simulink model "model1_visualize_video"  (R2025a)
settings: Solver=VariableStepAuto  StartTime=0.0  StopTime=10.0  RelTol=1e-3
settings Model: Creator=z004f2se  LastModifiedBy=z004f2se

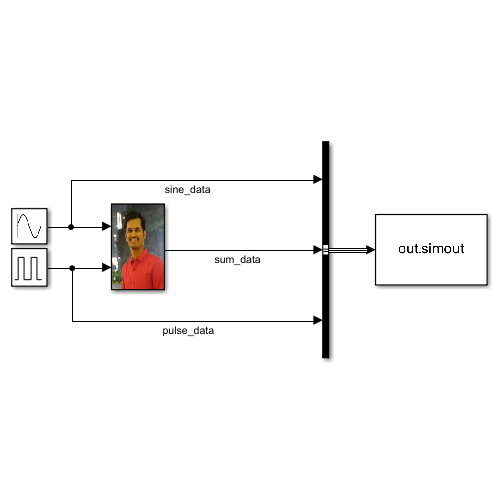
[thumbnail: Simulink's stored preview of the top-level diagram]
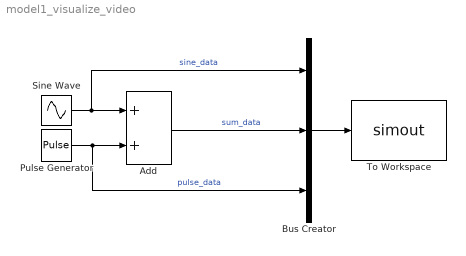
== system model1_visualize_video ==
  Add : Sum
      mask Display: image('VishalImage1.jpg');
  Bus Creator : BusCreator  Inputs=3
  Pulse Generator : DiscretePulseGenerator  PulseType=Time based  Period=10  PulseWidth=5
  Sine Wave : Sin  SampleTime=0
  To Workspace : ToWorkspace  VariableName=simout  SaveFormat=Timeseries  SampleTime=-1
  wires:
  Sine Wave/1 -> Bus Creator/1, Add/1  "sine_data"
  Pulse Generator/1 -> Bus Creator/3, Add/2  "pulse_data"
  Add/1 -> Bus Creator/2  "sum_data"
  Bus Creator/1 -> To Workspace/1
